simulink model "two_link_robot_dynamic_withoutg"  (R2020b)
settings: Solver=VariableStepAuto  StartTime=0.0  StopTime=10.0  RelTol=1e-3  EnableMultiTasking=on
undefined symbols (not defined in the file or in its folder): X, Y, Z
libraries: sm_lib x11, nesl_utility x11
settings Model: Creator=DELL  LastModifiedBy=Administrator
settings DataIOCC: LimitDataPoints=on  ReturnWorkspaceOutputs=off
settings OptimizationCC: LifeSpan=inf
settings DebuggingCC: AllowSymbolicDim=off  SFUnexpectedBacktrackingDiag=warning  SFNoUnconditionalDefaultTransitionDiag=warning  SFExecutionAtInitializationDiag=none  ArithmeticOperatorsInVariantConditions=warning
settings SFSimCC: SimUseLocalCustomCode=off  CustomCodeUndefinedFunction=UseInterfaceOnly
settings RTWCC: RTWUseLocalCustomCode=off
settings CodeAppCC: StateflowObjectComments=on
settings GRTTargetCC: TargetLangStandard=C89/C90 (ANSI)
settings ConfigComp: CovMetricSettings=dw  CovSaveCumulativeToWorkspaceVar=on  CovSaveSingleToWorkspaceVar=on  CovExternalEMLEnable=off  CovSFcnEnable=off
settings SimscapeCC: SimscapeNominalValues="[{\"value\":\"10\",\"unit\":\"V\"},{\"value\":\"1\",\"unit\":\"A\"},{\"value\":\"10\",\"unit\":\"N*m\"},{\"value\":\"10\",\"unit\":\"bar\"},{\"value\":\"100\",\"unit\":\"kJ/kg\"},{\"value\":\"1\",\"unit\":\"kW\"},{\"value\":\"300\",\"unit\":\"K\"},{\"value\":\"100\",\"unit\":\"cm^3/s\"},{\"value\":\"1\",\"unit\":\"kN\"},{\"value\":\"1\",\"unit\":\"g/cm^3\"},{\"value\":\"1\",\"unit\":\"l\"},{\"value\":\"1\",\"unit\":\"cm^2\"},{\"value\":\"60\",\"unit\":\"Hz\"}]"  SimscapeLogType=all  SimscapeLogDataHistory=10000
settings ConfigurationSet: Description=SimMechanics 2G

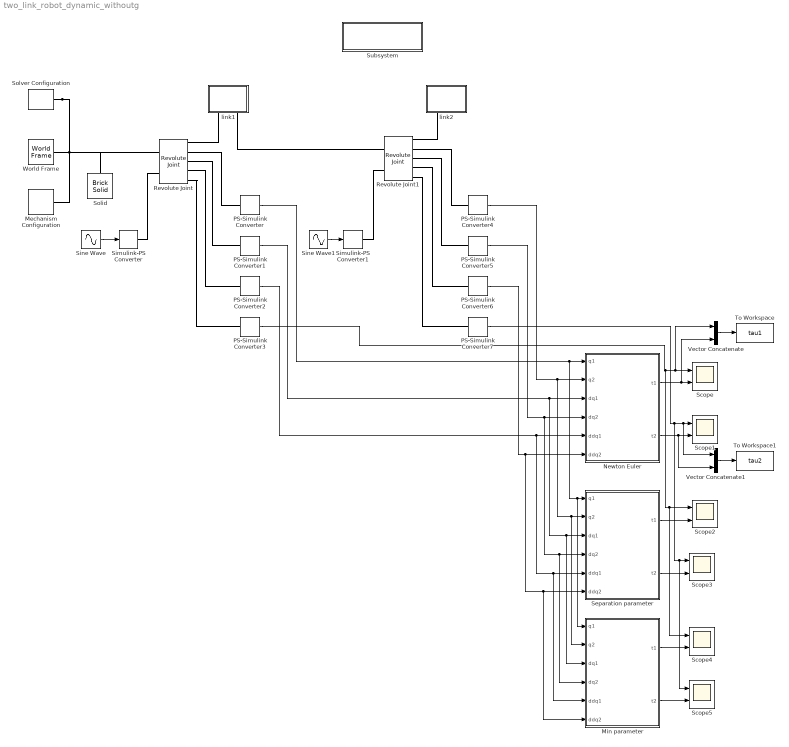
== system two_link_robot_dynamic_withoutg ==
  Mechanism Configuration : sm_lib/Utilities/Mechanism Configuration  UniformGravity=Constant  GravityVector=[0 0 0]  GravityVectorUnits=m/s^2  GravityUnits=m/s^2  LinearizationDelta=0.001  JointModeTransitionNonlinearIterations=2
  Min parameter : MATLAB Function  TreatAsAtomicUnit=on
  Newton Euler : MATLAB Function  TreatAsAtomicUnit=on
  PS-Simulink Converter{,1..7} (8 alike) : nesl_utility/PS-Simulink Converter  PhysicalDomain=network_engine_domain  SubClassName=ps_output  LeftPortType=input  RightPortType=output  PseudoPeriodic=off  Frequencies=[]  Unit=1  AffineConversion=off
  Revolute Joint : sm_lib/Joints/Revolute Joint  JointMode=Normal  SenseConstraintForce=off  SenseConstraintForceX=off  SenseConstraintForceY=off  SenseConstraintForceZ=off  SenseConstraintTorque=off  SenseConstraintTorqueX=off  SenseConstraintTorqueY=off  SenseConstraintTorqueZ=off  SenseTotalForce=off  SenseTotalForceX=off  SenseTotalForceY=off  SenseTotalForceZ=off  SenseTotalTorque=off  SenseTotalTorqueX=off  SenseTotalTorqueY=off  SenseTotalTorqueZ=off  CompositeWrenchDir=FollowerOnBase  CompositeWrenchFrame=BaseFrame  EquilibriumPosition=0  EquilibriumPositionUnits=deg  SpringStiffness=0  SpringStiffnessUnits=N*m/deg  DampingCoefficient=0  DampingCoefficientUnits=N*m/(deg/s)  TorqueActuationMode=ComputedTorque  MotionActuationMode=InputMotion  SensePosition=on  SenseVelocity=on  SenseAcceleration=on  SenseTorqueForce=on  SenseLowerLimitTorqueForce=off  SenseUpperLimitTorqueForce=off  LowerLimitSpecify=off  LowerLimitBound=-90  LowerLimitBoundUnits=deg  LowerLimitStiffness=1e4  LowerLimitStiffnessUnits=N*m/deg  LowerLimitDamping=10  LowerLimitDampingUnits=N*m/(deg/s)  LowerLimitTransitionRegionWidth=0.1  LowerLimitTransitionRegionWidthUnits=deg  UpperLimitSpecify=off  UpperLimitBound=90  UpperLimitBoundUnits=deg  UpperLimitStiffness=1e4  UpperLimitStiffnessUnits=N*m/deg  UpperLimitDamping=10  UpperLimitDampingUnits=N*m/(deg/s)  UpperLimitTransitionRegionWidth=0.1  UpperLimitTransitionRegionWidthUnits=deg  PositionTargetSpecify=off  PositionTargetPriority=High  PositionTargetValue=0  PositionTargetValueUnits=deg  VelocityTargetSpecify=off  VelocityTargetPriority=High  VelocityTargetValue=0  VelocityTargetValueUnits=deg/s
  Revolute Joint1 : sm_lib/Joints/Revolute Joint  JointMode=Normal  SenseConstraintForce=off  SenseConstraintForceX=off  SenseConstraintForceY=off  SenseConstraintForceZ=off  SenseConstraintTorque=off  SenseConstraintTorqueX=off  SenseConstraintTorqueY=off  SenseConstraintTorqueZ=off  SenseTotalForce=off  SenseTotalForceX=off  SenseTotalForceY=off  SenseTotalForceZ=off  SenseTotalTorque=off  SenseTotalTorqueX=off  SenseTotalTorqueY=off  SenseTotalTorqueZ=off  CompositeWrenchDir=FollowerOnBase  CompositeWrenchFrame=BaseFrame  EquilibriumPosition=0  EquilibriumPositionUnits=deg  SpringStiffness=0  SpringStiffnessUnits=N*m/deg  DampingCoefficient=0  DampingCoefficientUnits=N*m/(deg/s)  TorqueActuationMode=ComputedTorque  MotionActuationMode=InputMotion  SensePosition=on  SenseVelocity=on  SenseAcceleration=on  SenseTorqueForce=on  SenseLowerLimitTorqueForce=off  SenseUpperLimitTorqueForce=off  LowerLimitSpecify=off  LowerLimitBound=-90  LowerLimitBoundUnits=deg  LowerLimitStiffness=1e4  LowerLimitStiffnessUnits=N*m/deg  LowerLimitDamping=10  LowerLimitDampingUnits=N*m/(deg/s)  LowerLimitTransitionRegionWidth=0.1  LowerLimitTransitionRegionWidthUnits=deg  UpperLimitSpecify=off  UpperLimitBound=90  UpperLimitBoundUnits=deg  UpperLimitStiffness=1e4  UpperLimitStiffnessUnits=N*m/deg  UpperLimitDamping=10  UpperLimitDampingUnits=N*m/(deg/s)  UpperLimitTransitionRegionWidth=0.1  UpperLimitTransitionRegionWidthUnits=deg  PositionTargetSpecify=off  PositionTargetPriority=High  PositionTargetValue=0  PositionTargetValueUnits=deg  VelocityTargetSpecify=off  VelocityTargetPriority=High  VelocityTargetValue=0  VelocityTargetValueUnits=deg/s
  Scope{,1..5} (6 alike) : Scope  NumInputPorts=2
  Separation parameter : MATLAB Function  TreatAsAtomicUnit=on
  Simulink-PS Converter : nesl_utility/Simulink-PS Converter  PhysicalDomain=network_engine_domain  SubClassName=ps_input  LeftPortType=input  RightPortType=output  PseudoPeriodic=off  Frequencies=[]  NoiseDistribution=none  NoiseParameters=[]  Unit=1  AffineConversion=off  FilteringAndDerivatives=filter  SimscapeFilterOrder=2  InputFilterTimeConstant=0.001  UdotUserProvided=0
  Simulink-PS Converter1 : nesl_utility/Simulink-PS Converter  PhysicalDomain=network_engine_domain  SubClassName=ps_input  LeftPortType=input  RightPortType=output  PseudoPeriodic=off  Frequencies=[]  NoiseDistribution=none  NoiseParameters=[]  Unit=1  AffineConversion=off  FilteringAndDerivatives=filter  SimscapeFilterOrder=2  InputFilterTimeConstant=0.001  UdotUserProvided=0
  Sine Wave : Sin  Amplitude=2  Frequency=2  SampleTime=0
  Sine Wave1 : Sin  Frequency=3  SampleTime=0
  Solid : sm_lib/Body Elements/Brick Solid  GraphicAmbientColor=[0.15 0.15 0.15 1.0]  BasedOnType=Density  BrickDimensions=[0.04 0.04 0.04]  BrickDimensionUnits=m  CenterOfMass=[0 0 0]  CenterOfMassUnits=m  GraphicDiffuseColor=[0.85 0.45 0]  Density=1000  DensityUnits=kg/m^3  DoExposeReferenceFrame=on  GraphicEmissiveColor=[0.0 0.0 0.0 1.0]  ExportEntireGeometry=off  SerializedFrames=<Frames/>  MarkerShape=Sphere  MarkerSize=10  GraphicType=FromGeometry  InertiaType=CalculateFromGeometry  Mass=1  MassUnits=kg  MomentsOfInertia=[1 1 1]  MomentsOfInertiaUnits=kg*m^2  GraphicOpacity=1.0  ProductsOfInertia=[0 0 0]  ProductsOfInertiaUnits=kg*m^2  GraphicShininess=75  GraphicSpecularColor=[0.5 0.5 0.5 1.0]  GraphicVisPropType=SimpleVisualProperties
  Solver Configuration : nesl_utility/Solver Configuration  PhysicalDomain=network_engine_domain  SubClassName=solver  LeftPortType=input  RightPortType=generic  Tones=[]  Harmonics=[]  SimulateNoise=off  Profile=off  UseLocalSampling=off  EnableSwitchedLinearOptims=on  FrequencyDomain=off  UseCCode=off  RelTol=0.001  AbsTol=1e-06  MinStep=1e-09  ToWorkspace=off  RevertToSquareIcSolve=off  NumHomotopyIterations=100  PhasorMode=off  PhasorModeNumHarmonics=1  DoDC=off  ResidualTolerance=1e-09  UseLocalSolver=off  LocalSolverChoice=NE_BACKWARD_EULER_ADVANCER  LocalSolverSampleTime=0.001  DoFixedCost=off  MaxNonlinIter=3  MaxModeIter=2  ComputeImpulses=off  ImpulseIterations=2  LinearAlgebra=Sparse  EquationFormulation=NE_TIME_EF  DelaysMemoryBudget=1024  AutomaticFiltering=on  FilteringTimeConstant=0.001  PartitionStorageMethod=AS_NEEDED  PartitionMemoryBudget=1024  PartitionMethod=FAST
  Subsystem : Subsystem
      settings: OpenFcn=open_system('sm_lib')
      mask Display: disp(sprintf('Open Simscape Multibody\nLibrary'));
  To Workspace : ToWorkspace  VariableName=tau1  SaveFormat=Timeseries  SampleTime=-1
  To Workspace1 : ToWorkspace  VariableName=tau2  SaveFormat=Timeseries  SampleTime=-1
  Vector Concatenate : Concatenate
  Vector Concatenate1 : Concatenate
  World Frame : sm_lib/Frames and Transforms/World Frame
  link1 : Subsystem  mask{r=0.01, l=0.3, rho=100000000, rgb=[0.2, 0.2, 0.8]}
      mask prompts: r "radius(m)"; l "length(m)"; rho "density(kg/m^3)"; rgb "Color[R G B]"
  link2 : Subsystem  mask{r=0.01, l=0.2, rho=200000000, rgb=[0.2, 0.2, 0.8]}
      mask prompts: r "radius(m)"; l "length(m)"; rho "density(kg/m^3)"; rgb "Color[R G B]"
  wires:
  Sine Wave/1 -> Simulink-PS Converter/1
  Sine Wave1/1 -> Simulink-PS Converter1/1
  PS-Simulink Converter/1 -> Min parameter/1(q1), Separation parameter/1(q1), Newton Euler/1(q1)
  PS-Simulink Converter4/1 -> Min parameter/2(q2), Separation parameter/2(q2), Newton Euler/2(q2)
  PS-Simulink Converter1/1 -> Min parameter/3(dq1), Separation parameter/3(dq1), Newton Euler/3(dq1)
  PS-Simulink Converter5/1 -> Min parameter/4(dq2), Separation parameter/4(dq2), Newton Euler/4(dq2)
  PS-Simulink Converter2/1 -> Min parameter/5(ddq1), Separation parameter/5(ddq1), Newton Euler/5(ddq1)
  PS-Simulink Converter6/1 -> Min parameter/6(ddq2), Separation parameter/6(ddq2), Newton Euler/6(ddq2)
  Newton Euler/1(t1) -> Vector Concatenate/2, Scope/2
  PS-Simulink Converter3/1 -> Scope4/1, Scope2/1, Vector Concatenate/1, Scope/1
  Newton Euler/2(t2) -> Scope1/2, Vector Concatenate1/2
  PS-Simulink Converter7/1 -> Scope5/1, Scope3/1, Vector Concatenate1/1, Scope1/1
  Vector Concatenate/1 -> To Workspace/1
  Vector Concatenate1/1 -> To Workspace1/1
  Separation parameter/1(t1) -> Scope2/2
  Separation parameter/2(t2) -> Scope3/2
  Min parameter/1(t1) -> Scope4/2
  Min parameter/2(t2) -> Scope5/2
  connections:
  Solver Configuration/RConn1 -- Solid/RConn1 -- Revolute Joint/LConn1 -- Mechanism Configuration/RConn1 -- World Frame/RConn1
  link1/RConn1 -- Revolute Joint/RConn1
  link1/RConn2 -- Revolute Joint1/LConn1
  Revolute Joint1/RConn1 -- link2/RConn1
  Simulink-PS Converter/RConn1 -- Revolute Joint/LConn2
  Simulink-PS Converter1/RConn1 -- Revolute Joint1/LConn2
  Revolute Joint/RConn2 -- PS-Simulink Converter/LConn1
  Revolute Joint/RConn3 -- PS-Simulink Converter1/LConn1
  Revolute Joint/RConn4 -- PS-Simulink Converter2/LConn1
  Revolute Joint/RConn5 -- PS-Simulink Converter3/LConn1
  Revolute Joint1/RConn2 -- PS-Simulink Converter4/LConn1
  Revolute Joint1/RConn3 -- PS-Simulink Converter5/LConn1
  Revolute Joint1/RConn4 -- PS-Simulink Converter6/LConn1
  Revolute Joint1/RConn5 -- PS-Simulink Converter7/LConn1

== system two_link_robot_dynamic_withoutg/Subsystem ==

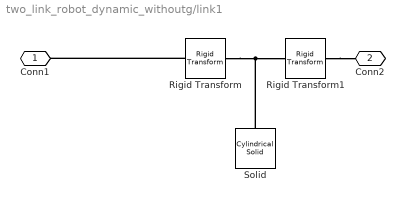
== system two_link_robot_dynamic_withoutg/link1 ==
  Rigid Transform : sm_lib/Frames and Transforms/Rigid Transform  TranslationMethod=StandardAxis  TranslationStandardOffset=l/2  TranslationLengthUnit=m  TranslationStandardAxis=-X  TranslationCartesianOffset=[0 0 0]  TranslationROffset=0  TranslationROffsetUnits=m  TranslationZOffset=0  TranslationZOffsetUnits=m  TranslationThetaOffset=0  TranslationThetaOffsetUnits=deg  RotationMethod=None  RotationAngleUnits=deg  RotationStandardAxis=-X  RotationAngle=0.0  RotationArbitraryAxis=[0 0 1]  FollAlignAxisA=+X  BaseAlignAxisA=+Y  FollAlignAxisB=+Y  BaseAlignAxisB=+Z  RotationSequenceAxes=FollowerAxes  RotationSequence=XYX  RotationSequenceAngles=[0 0 0]  RotationSequenceAnglesUnits=deg  RotationMatrix=[1 0 0; 0 1 0; 0 0 1]
  Rigid Transform1 : sm_lib/Frames and Transforms/Rigid Transform  TranslationMethod=StandardAxis  TranslationStandardOffset=l/2  TranslationLengthUnit=m  TranslationStandardAxis=+X  TranslationCartesianOffset=[0 0 0]  TranslationROffset=0  TranslationROffsetUnits=m  TranslationZOffset=0  TranslationZOffsetUnits=m  TranslationThetaOffset=0  TranslationThetaOffsetUnits=deg  RotationMethod=None  RotationAngleUnits=deg  RotationStandardAxis=+Z  RotationAngle=0.0  RotationArbitraryAxis=[0 0 1]  FollAlignAxisA=+X  BaseAlignAxisA=+Y  FollAlignAxisB=+Y  BaseAlignAxisB=+Z  RotationSequenceAxes=FollowerAxes  RotationSequence=XYX  RotationSequenceAngles=[0 0 0]  RotationSequenceAnglesUnits=deg  RotationMatrix=[1 0 0; 0 1 0; 0 0 1]
  Solid : sm_lib/Body Elements/Cylindrical Solid  GraphicAmbientColor=[0.15 0.15 0.15 1.0]  BasedOnType=Density  CenterOfMass=[0 0 0]  CenterOfMassUnits=m  GraphicDiffuseColor=rgb  CylinderLength=l  CylinderLengthUnits=m  CylinderRadius=r  CylinderRadiusUnits=m  Density=rho  DensityUnits=kg/m^3  DoExposeReferenceFrame=off  GraphicEmissiveColor=[0.0 0.0 0.0 1.0]  ExportEntireGeometry=off  SerializedFrames=<Frames><Frame><Id>Frame1</Id><Value><Name>F1</Name><Origin><Source>ReferenceFrame</Source><FeatureName></FeatureName></Origin><PrimaryAxis><DefinedDirection>+X</DefinedDirection><Source>ReferenceFrame</Source><SourceDirection>+Z</SourceDirection><FeatureName></FeatureName></PrimaryAxis><SecondaryAxis><DefinedDirection>+Y</DefinedDirection><Source>ReferenceFrame</Source><SourceDirection>+X</SourceDirection><FeatureName></FeatureName></SecondaryAxis></Value></Frame></Frames>  MarkerShape=Sphere  MarkerSize=10  GraphicType=FromGeometry  InertiaType=CalculateFromGeometry  Mass=1  MassUnits=kg  MomentsOfInertia=[1 1 1]  MomentsOfInertiaUnits=kg*m^2  GraphicOpacity=1.0  ProductsOfInertia=[0 0 0]  ProductsOfInertiaUnits=kg*m^2  GraphicShininess=75  GraphicSpecularColor=[0.5 0.5 0.5 1.0]  GraphicVisPropType=SimpleVisualProperties
  Conn1 : PMIOPort  Side=Right
  Conn2 : PMIOPort  Port=2  Side=Right
  connections:
  Rigid Transform/LConn1 -- Rigid Transform1/LConn1 -- Solid/LConn1
  Rigid Transform1/RConn1 -- Conn2/RConn1
  Rigid Transform/RConn1 -- Conn1/RConn1

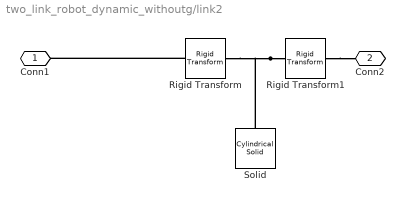
== system two_link_robot_dynamic_withoutg/link2 ==
  Rigid Transform : sm_lib/Frames and Transforms/Rigid Transform  TranslationMethod=StandardAxis  TranslationStandardOffset=l/2  TranslationLengthUnit=m  TranslationStandardAxis=-X  TranslationCartesianOffset=[0 0 0]  TranslationROffset=0  TranslationROffsetUnits=m  TranslationZOffset=0  TranslationZOffsetUnits=m  TranslationThetaOffset=0  TranslationThetaOffsetUnits=deg  RotationMethod=None  RotationAngleUnits=deg  RotationStandardAxis=-X  RotationAngle=0.0  RotationArbitraryAxis=[0 0 1]  FollAlignAxisA=+X  BaseAlignAxisA=+Y  FollAlignAxisB=+Y  BaseAlignAxisB=+Z  RotationSequenceAxes=FollowerAxes  RotationSequence=XYX  RotationSequenceAngles=[0 0 0]  RotationSequenceAnglesUnits=deg  RotationMatrix=[1 0 0; 0 1 0; 0 0 1]
  Rigid Transform1 : sm_lib/Frames and Transforms/Rigid Transform  TranslationMethod=StandardAxis  TranslationStandardOffset=l/2  TranslationLengthUnit=m  TranslationStandardAxis=+X  TranslationCartesianOffset=[0 0 0]  TranslationROffset=0  TranslationROffsetUnits=m  TranslationZOffset=0  TranslationZOffsetUnits=m  TranslationThetaOffset=0  TranslationThetaOffsetUnits=deg  RotationMethod=None  RotationAngleUnits=deg  RotationStandardAxis=+Z  RotationAngle=0.0  RotationArbitraryAxis=[0 0 1]  FollAlignAxisA=+X  BaseAlignAxisA=+Y  FollAlignAxisB=+Y  BaseAlignAxisB=+Z  RotationSequenceAxes=FollowerAxes  RotationSequence=XYX  RotationSequenceAngles=[0 0 0]  RotationSequenceAnglesUnits=deg  RotationMatrix=[1 0 0; 0 1 0; 0 0 1]
  Solid : sm_lib/Body Elements/Cylindrical Solid  GraphicAmbientColor=[0.15 0.15 0.15 1.0]  BasedOnType=Density  CenterOfMass=[0 0 0]  CenterOfMassUnits=m  GraphicDiffuseColor=rgb  CylinderLength=l  CylinderLengthUnits=m  CylinderRadius=r  CylinderRadiusUnits=m  Density=rho  DensityUnits=kg/m^3  DoExposeReferenceFrame=off  GraphicEmissiveColor=[0.0 0.0 0.0 1.0]  ExportEntireGeometry=off  SerializedFrames=<Frames><Frame><Id>Frame1</Id><Value><Name>F1</Name><Origin><Source>ReferenceFrame</Source><FeatureName></FeatureName></Origin><PrimaryAxis><DefinedDirection>+X</DefinedDirection><Source>ReferenceFrame</Source><SourceDirection>+Z</SourceDirection><FeatureName></FeatureName></PrimaryAxis><SecondaryAxis><DefinedDirection>+Y</DefinedDirection><Source>ReferenceFrame</Source><SourceDirection>+X</SourceDirection><FeatureName></FeatureName></SecondaryAxis></Value></Frame></Frames>  MarkerShape=Sphere  MarkerSize=10  GraphicType=FromGeometry  InertiaType=CalculateFromGeometry  Mass=1  MassUnits=kg  MomentsOfInertia=[1 1 1]  MomentsOfInertiaUnits=kg*m^2  GraphicOpacity=1.0  ProductsOfInertia=[0 0 0]  ProductsOfInertiaUnits=kg*m^2  GraphicShininess=75  GraphicSpecularColor=[0.5 0.5 0.5 1.0]  GraphicVisPropType=SimpleVisualProperties
  Conn1 : PMIOPort  Side=Right
  Conn2 : PMIOPort  Port=2  Side=Right
  connections:
  Rigid Transform/RConn1 -- Conn1/RConn1
  Rigid Transform1/RConn1 -- Conn2/RConn1
  Rigid Transform1/LConn1 -- Rigid Transform/LConn1 -- Solid/LConn1

== matlab function two_link_robot_dynamic_withoutg/Separation parameter ==
  data: q1 input; t1 output; q2 input; dq1 input; dq2 input; ddq1 input; ddq2 input; t2 output
function [t1,t2] = fcn(q1,q2,dq1,dq2,ddq1,ddq2)
%连杆1质心惯性张量
L_1xx = 0.471239;
L_1xy = 0;
L_1xz = 0;
L_1yy = 70.9215;
L_1yz = 0;
L_1zz = 70.9215;
m_1 = 9424.78;
L_1c = [L_1xx 0 0;0 L_1yy 0;0 0 L_1zz];
%连杆2质心惯性张量
L_2xx = 0.628319;
L_2xy = 0;
L_2xz = 0;
L_2yy = 42.2021;
L_2yz = 0;
L_2zz = 42.2021;
m_2 = 12566.4;
L_2c = [L_2xx 0 0;0 L_2yy 0;0 0 L_2zz];
%连杆长度
l1 = 0.3;
l2 = 0.2;
%质心坐标
l_1x = l1 / 2;
l_1y = 0;
l_1z = 0;
pc1 = [l_1x l_1y l_1z]';
l_2x = l2 / 2;
l_2y = 0;
l_2z = 0;
pc2 = [l_2x l_2y l_2z]';
%平行轴定理，旋转轴处的惯性张量
I3 = eye(3);
L_1 = L_1c + m_1*(pc1'*pc1*I3 - pc1*pc1');
L_2 = L_2c + m_2*(pc2'*pc2*I3 - pc2*pc2');

% 地杆角速度
w_0_0 = [0;0;0];
% 地杆线速度速度
v_0_0 = [0;0;0];
% angular acceleration of base link
alpha_0_0 = [0; 0; 0];
% 考虑重力，初始加速度y0方向
% a_0_0 = [0; 9.81; 0];
a_0_0 = [0; 0; 0];

dh = [0, 0, 0, q1;
      0, l1, 0, q2];

w = cell(1, size(dh, 1));
v = cell(1, size(dh, 1));
alpha = cell(1, size(dh, 1));
a = cell(1, size(dh, 1));
ac = cell(1, size(dh, 1));
l = cell(1, size(dh, 1));
T = cell(1, size(dh, 1) + 1);
R = cell(1, size(dh, 1) + 1);
r = cell(1, size(dh, 1) + 1);
I = cell(1, size(dh, 1));
T_e = cell(1, size(dh, 1) + 1);
t_e_pre = eye(4);
for i = 1:size(dh, 1)
    trx = [1 0 0 0; 
           0 cos(dh(i, 1)) -sin(dh(i, 1)) 0;
           0 sin(dh(i, 1)) cos(dh(i, 1))  0;
           0 0 0 1];
    tl = [1 0 0 dh(i, 2);
          0 1 0 0;
          0 0 1 dh(i, 3);
          0 0 0 1];
    trz = [cos(dh(i, 4)) -sin(dh(i, 4)) 0 0;
           sin(dh(i, 4)) cos(dh(i, 4))  0 0;
           0 0 1 0;
           0 0 0 1];
    T{i} = trx * tl * trz;%trotx(dh(i, 1))*transl([dh(i, 2), 0, dh(i, 3)])*trotz(dh(i, 4));
    R{i} = T{i}(1:3, 1:3);
    r{i} = T{i}(1:3, 4);
    T_e{i} = t_e_pre * T{i};
    t_e_pre = T_e{i};
end
T{i+1} = eye(3);
R{i+1} = eye(3);
r{i+1} = [l2, 0, 0];
T_e{i+1} = T_e{i} * [1 0 0 l2; 0 1 0 0; 0 0 1 0; 0 0 0 1];%T_e{i} * transl([l2, 0, 0]);
q = [q1 q2];
dq = [dq1 dq2];
ddq = [ddq1 ddq2];
l{1} = [l_1x; l_1y; l_1z];
l{2} = [l_2x; l_2y; l_2z];

pre_w = w_0_0;
pre_v = v_0_0;
pre_alpha = alpha_0_0;
pre_a = a_0_0;
% 外推
for i = 1:2
    t = R{i}';
    w_i_i = t * pre_w + dq(i) * [0;0;1];
    v_i_i = t * (pre_v + cross(pre_w, r{i}));
    alpha_i_i = t * pre_alpha + cross((t * pre_w), dq(i) * [0;0;1]) + ddq(i) * [0;0;1];
    a_i_i = t * (pre_a + cross(pre_alpha, r{i}) + cross(pre_w, cross(pre_w, r{i})));
    ac_i_i = a_i_i + cross(alpha_i_i, l{i}) + cross(w_i_i, cross(w_i_i, l{i}));
    w{i} = w_i_i;
    v{i} = v_i_i;
    alpha{i} = alpha_i_i;
    a{i} = a_i_i;
    ac{i} = ac_i_i;
    
    pre_w = w_i_i;
    pre_v = v_i_i;
    pre_alpha = alpha_i_i;
    pre_a = a_i_i;
end

%参数分离参数
A1 = zeros(6,10);
A2 = zeros(6,10);
A1(1:3,1) = a{1};
A1(1:3,2:4) = S_alg(alpha{1})+S_alg(w{1})*S_alg(w{1});
A1(4:6,2:4) = -S_alg(a{1});
A1(4:6,5:10) = K_alg(alpha{1})+S_alg(w{1})*K_alg(w{1});
A2(1:3,1) = a{2};
A2(1:3,2:4) = S_alg(alpha{2})+S_alg(w{2})*S_alg(w{2});
A2(4:6,2:4) = -S_alg(a{2});
A2(4:6,5:10) = K_alg(alpha{2})+S_alg(w{2})*K_alg(w{2});

R21 = R{2};
P21 = r{2};
Q12 = [R21 zeros(3,3);S_alg(P21)*R21 R21];
U11 = A1;
U12 = Q12*A2;
U22 = A2; 
U1 = [U11 U12;
zeros(6,10) U22]; 
U = [U1(6,:);
 U1(12,:);]; 
%     
fi1 = [m_1 m_1*l_1x m_1*l_1y m_1*l_1z L_1(1,1) -L_1(1,2) -L_1(1,3) L_1(2,2) -L_1(2,3) L_1(3,3)]';
fi2  = [m_2 m_2*l_2x m_2*l_2y m_2*l_2z L_2(1,1) -L_2(1,2) -L_2(1,3) L_2(2,2) -L_2(2,3) L_2(3,3)]';
fi = [fi1;fi2]; %线性分离的  
f = U1*fi;
t1 = f(6);
t2 = f(12);
end

function T = K_alg(w)
 wx = w(1);wy = w(2);wz = w(3);
 T = zeros(3,6);
 T(1,1) = wx;T(1,2) = wy;T(1,3) = wz;
 T(2,2) = wx;T(2,4) = wy;T(2,5) = wz;
 T(3,3) = wx;T(3,5) = wy;T(3,6) = wz;
end

function T = S_alg(w)
 w_r = eye(3);
 A1 = w(1);A2 = w(2);A3 = w(3);
 w_r(1,1) = 0;w_r(1,2) = -A3;w_r(1,3) = A2;
 w_r(2,1) = A3;w_r(2,2) = 0;w_r(2,3) = -A1;
 w_r(3,1) = -A2;w_r(3,2) = A1;w_r(3,3) = 0;
 T = w_r;
end

== matlab function two_link_robot_dynamic_withoutg/Newton Euler ==
  data: q1 input; t1 output; q2 input; dq1 input; dq2 input; ddq1 input; ddq2 input; t2 output
function [t1,t2] = fcn(q1,q2,dq1,dq2,ddq1,ddq2)
%连杆1质心惯性张量
L_1xx = 0.471239;
L_1xy = 0;
L_1xz = 0;
L_1yy = 70.9215;
L_1yz = 0;
L_1zz = 70.9215;
m_1 = 9424.78;
L_1c = [L_1xx 0 0;0 L_1yy 0;0 0 L_1zz];
%连杆2质心惯性张量
L_2xx = 0.628319;
L_2xy = 0;
L_2xz = 0;
L_2yy = 42.2021;
L_2yz = 0;
L_2zz = 42.2021;
m_2 = 12566.4;
L_2c = [L_2xx 0 0;0 L_2yy 0;0 0 L_2zz];
%连杆长度
l1 = 0.3;
l2 = 0.2;
%质心坐标
l_1x = l1 / 2;
l_1y = 0;
l_1z = 0;
pc1 = [l_1x l_1y l_1z]';
l_2x = l2 / 2;
l_2y = 0;
l_2z = 0;
pc2 = [l_2x l_2y l_2z]';
%平行轴定理，旋转轴处的惯性张量
I3 = eye(3);
L_1 = L_1c + m_1*(pc1'*pc1*I3 - pc1*pc1');
L_2 = L_2c + m_2*(pc2'*pc2*I3 - pc2*pc2');

% 地杆角速度
w_0_0 = [0;0;0];
% 地杆线速度速度
v_0_0 = [0;0;0];
% angular acceleration of base link
alpha_0_0 = [0; 0; 0];
% 不考虑重力
% a_0_0 = [0; 9.81; 0];
a_0_0 = [0; 0; 0];

dh = [0, 0, 0, q1;
      0, l1, 0, q2];

w = cell(1, size(dh, 1));
v = cell(1, size(dh, 1));
alpha = cell(1, size(dh, 1));
a = cell(1, size(dh, 1));
ac = cell(1, size(dh, 1));
l = cell(1, size(dh, 1));
T = cell(1, size(dh, 1) + 1);
R = cell(1, size(dh, 1) + 1);
r = cell(1, size(dh, 1) + 1);
I = cell(1, size(dh, 1));
T_e = cell(1, size(dh, 1) + 1);
t_e_pre = eye(4);
for i = 1:size(dh, 1)
    trx = [1 0 0 0; 
           0 cos(dh(i, 1)) -sin(dh(i, 1)) 0;
           0 sin(dh(i, 1)) cos(dh(i, 1))  0;
           0 0 0 1];
    tl = [1 0 0 dh(i, 2);
          0 1 0 0;
          0 0 1 dh(i, 3);
          0 0 0 1];
    trz = [cos(dh(i, 4)) -sin(dh(i, 4)) 0 0;
           sin(dh(i, 4)) cos(dh(i, 4))  0 0;
           0 0 1 0;
           0 0 0 1];
    T{i} = trx * tl * trz;%trotx(dh(i, 1))*transl([dh(i, 2), 0, dh(i, 3)])*trotz(dh(i, 4));其次变换矩阵
    R{i} = T{i}(1:3, 1:3);
    r{i} = T{i}(1:3, 4);
    T_e{i} = t_e_pre * T{i};
    t_e_pre = T_e{i};
end
T{i+1} = eye(3);
R{i+1} = eye(3);
r{i+1} = [l2, 0, 0];
T_e{i+1} = T_e{i} * [1 0 0 l2; 0 1 0 0; 0 0 1 0; 0 0 0 1];%T_e{i} * transl([l2, 0, 0]);
q = [q1 q2];
dq = [dq1 dq2];
ddq = [ddq1 ddq2];
l{1} = [l_1x; l_1y; l_1z];
l{2} = [l_2x; l_2y; l_2z];

pre_w = w_0_0;
pre_v = v_0_0;
pre_alpha = alpha_0_0;
pre_a = a_0_0;
% 外推
for i = 1:2
    t = R{i}';
    w_i_i = t * pre_w + dq(i) * [0;0;1];
    v_i_i = t * (pre_v + cross(pre_w, r{i}));
    alpha_i_i = t * pre_alpha + cross((t * pre_w), dq(i) * [0;0;1]) + ddq(i) * [0;0;1];
    a_i_i = t * (pre_a + cross(pre_alpha, r{i}) + cross(pre_w, cross(pre_w, r{i})));
    ac_i_i = a_i_i + cross(alpha_i_i, l{i}) + cross(w_i_i, cross(w_i_i, l{i}));
    w{i} = w_i_i;
    v{i} = v_i_i;
    alpha{i} = alpha_i_i;
    a{i} = a_i_i;
    ac{i} = ac_i_i;
    
    pre_w = w_i_i;
    pre_v = v_i_i;
    pre_alpha = alpha_i_i;
    pre_a = a_i_i;
end
m = [m_1; m_2];
% 内推
f_3_3 = [0;0;0];
n_3_3 = [0;0;0];
next_f_i_i = f_3_3;
next_n_i_i = n_3_3;

I{1} = [L_1xx L_1xy L_1xz; L_1xy L_1yy L_1yz; L_1xz L_1yz L_1zz];
I{2} = [L_2xx L_2xy L_2xz; L_2xy L_2yy L_2yz; L_2xz L_2yz L_2zz];
tau = cell(1, size(dh, 1));

for i = 2:-1:1
    rr = R{i+1};
    f_i_i = m(i)*ac{i} + rr * next_f_i_i;
    
    TT = T_e{i};
    TT(1:3,1:3) = (T_e{i}(1:3,1:3))';
    TT(1:3, 4) = -(T_e{i}(1:3,1:3))' * T_e{i}(1:3,4);
    xx = TT * T_e{i+1}(1:4, 4);
    r_ip1_ci = l{i} - xx(1:3);
    torque_i = I{i}*alpha{i} + cross(w{i}, I{i}*w{i}) + rr * next_n_i_i + cross(l{i}, f_i_i) - cross(r_ip1_ci, rr * next_f_i_i);
    tau{i} = torque_i(3);
    next_f_i_i = f_i_i;
    next_n_i_i = torque_i;
end
t1 = tau{1};
t2 = tau{2};


end

== matlab function two_link_robot_dynamic_withoutg/Min parameter ==
  data: q1 input; t1 output; q2 input; dq1 input; dq2 input; ddq1 input; ddq2 input; t2 output
function [t1,t2] = fcn(q1,q2,dq1,dq2,ddq1,ddq2)
%连杆1质心惯性张量
L_1xx = 0.471239;
L_1xy = 0;
L_1xz = 0;
L_1yy = 70.9215;
L_1yz = 0;
L_1zz = 70.9215;
m_1 = 9424.78;
L_1c = [L_1xx 0 0;0 L_1yy 0;0 0 L_1zz];
%连杆2质心惯性张量
L_2xx = 0.628319;
L_2xy = 0;
L_2xz = 0;
L_2yy = 42.2021;
L_2yz = 0;
L_2zz = 42.2021;
m_2 = 12566.4;
L_2c = [L_2xx 0 0;0 L_2yy 0;0 0 L_2zz];
%连杆长度
l1 = 0.3;
l2 = 0.2;
%质心坐标
l_1x = l1 / 2;
l_1y = 0;
l_1z = 0;
pc1 = [l_1x l_1y l_1z]';
l_2x = l2 / 2;
l_2y = 0;
l_2z = 0;
pc2 = [l_2x l_2y l_2z]';
%平行轴定理，旋转轴处的惯性张量
I3 = eye(3);
L_1 = L_1c + m_1*(pc1'*pc1*I3 - pc1*pc1');
L_2 = L_2c + m_2*(pc2'*pc2*I3 - pc2*pc2');

% 地杆角速度
w_0_0 = [0;0;0];
% 地杆线速度速度
v_0_0 = [0;0;0];
% angular acceleration of base link
alpha_0_0 = [0; 0; 0];
% 不考虑重力
% a_0_0 = [0; 9.81; 0];
a_0_0 = [0; 0; 0];

dh = [0, 0, 0, q1;
      0, l1, 0, q2];

w = cell(1, size(dh, 1));
v = cell(1, size(dh, 1));
alpha = cell(1, size(dh, 1));
a = cell(1, size(dh, 1));
ac = cell(1, size(dh, 1));
l = cell(1, size(dh, 1));
T = cell(1, size(dh, 1) + 1);
R = cell(1, size(dh, 1) + 1);
r = cell(1, size(dh, 1) + 1);
I = cell(1, size(dh, 1));
T_e = cell(1, size(dh, 1) + 1);
t_e_pre = eye(4);
for i = 1:size(dh, 1)
    trx = [1 0 0 0; 
           0 cos(dh(i, 1)) -sin(dh(i, 1)) 0;
           0 sin(dh(i, 1)) cos(dh(i, 1))  0;
           0 0 0 1];
    tl = [1 0 0 dh(i, 2);
          0 1 0 0;
          0 0 1 dh(i, 3);
          0 0 0 1];
    trz = [cos(dh(i, 4)) -sin(dh(i, 4)) 0 0;
           sin(dh(i, 4)) cos(dh(i, 4))  0 0;
           0 0 1 0;
           0 0 0 1];
    T{i} = trx * tl * trz;%trotx(dh(i, 1))*transl([dh(i, 2), 0, dh(i, 3)])*trotz(dh(i, 4));其次变换矩阵
    R{i} = T{i}(1:3, 1:3);
    r{i} = T{i}(1:3, 4);
    T_e{i} = t_e_pre * T{i};
    t_e_pre = T_e{i};
end
T{i+1} = eye(3);
R{i+1} = eye(3);
r{i+1} = [l2, 0, 0];
T_e{i+1} = T_e{i} * [1 0 0 l2; 0 1 0 0; 0 0 1 0; 0 0 0 1];%T_e{i} * transl([l2, 0, 0]);
q = [q1 q2];
dq = [dq1 dq2];
ddq = [ddq1 ddq2];
l{1} = [l_1x; l_1y; l_1z];
l{2} = [l_2x; l_2y; l_2z];

pre_w = w_0_0;
pre_v = v_0_0;
pre_alpha = alpha_0_0;
pre_a = a_0_0;
% 外推
for i = 1:2
    t = R{i}';
    w_i_i = t * pre_w + dq(i) * [0;0;1];
    v_i_i = t * (pre_v + cross(pre_w, r{i}));
    alpha_i_i = t * pre_alpha + cross((t * pre_w), dq(i) * [0;0;1]) + ddq(i) * [0;0;1];
    a_i_i = t * (pre_a + cross(pre_alpha, r{i}) + cross(pre_w, cross(pre_w, r{i})));
    ac_i_i = a_i_i + cross(alpha_i_i, l{i}) + cross(w_i_i, cross(w_i_i, l{i}));
    w{i} = w_i_i;
    v{i} = v_i_i;
    alpha{i} = alpha_i_i;
    a{i} = a_i_i;
    ac{i} = ac_i_i;
    
    pre_w = w_i_i;
    pre_v = v_i_i;
    pre_alpha = alpha_i_i;
    pre_a = a_i_i;
end

%参数分离参数
A1 = zeros(6,10);
A2 = zeros(6,10);
A1(1:3,1) = a{1};
A1(1:3,2:4) = S_alg(alpha{1})+S_alg(w{1})*S_alg(w{1});
A1(4:6,2:4) = -S_alg(a{1});
A1(4:6,5:10) = K_alg(alpha{1})+S_alg(w{1})*K_alg(w{1});
A2(1:3,1) = a{2};
A2(1:3,2:4) = S_alg(alpha{2})+S_alg(w{2})*S_alg(w{2});
A2(4:6,2:4) = -S_alg(a{2});
A2(4:6,5:10) = K_alg(alpha{2})+S_alg(w{2})*K_alg(w{2});

R21 = R{2};
P21 = r{2};
Q12 = [R21 zeros(3,3);S_alg(P21)*R21 R21];
U11 = A1;
U12 = Q12*A2;
U22 = A2; 
U1 = [U11 U12;
zeros(6,10) U22]; 
U = [U1(6,:);
 U1(12,:);]; 
    
fi1 = [m_1 m_1*l_1x m_1*l_1y m_1*l_1z L_1(1,1) -L_1(1,2) -L_1(1,3) L_1(2,2) -L_1(2,3) L_1(3,3)]';
fi2  = [m_2 m_2*l_2x m_2*l_2y m_2*l_2z L_2(1,1) -L_2(1,2) -L_2(1,3) L_2(2,2) -L_2(2,3) L_2(3,3)]';
%init
M2 = fi2(1,1);
MX2 = fi2(2,1);
MY2 = fi2(3,1);
MZ2 = fi2(4,1);
XX2 = fi2(5,1);
XY2 = fi2(6,1);
XZ2 = fi2(7,1);
YY2 = fi2(8,1);
YZ2 = fi2(9,1);
ZZ2 = fi2(10,1);
%r2
fi2_min_param = [MX2 MY2 ZZ2]';

d2 = 0;
a2 = l1;
alpha2 = 0;
cs2 = cos(alpha2)*sin(alpha2);
s2 = sin(alpha2);
c2 = cos(alpha2);

XX1 = fi1(5,1) + d2^2*M2;
XY1 = fi1(6,1) + a2*d2*s2*M2;
XZ1 = fi1(7,1) - a2*d2*c2*M2;
YY1 = fi1(8,1) + (a2^2 + d2^2*c2^2)*M2;
YZ1 = fi1(9,1) + d2^2*cs2*M2; 
ZZ1 = fi1(10,1) + (a2^2 + d2^2*s2^2)*M2;
MX1 = fi1(2,1) + a2*M2;
MY1 = fi1(3,1) - d2*s2*M2;
MZ1 = fi1(4,1) + d2*c2*M2;
M1 = fi1(1,1) + M2;

%r3
%不考虑重力
% fi1_min_param = [MX1 ZZ1]';
fi1_min_param =  ZZ1;
fi_min_param = [fi1_min_param;fi2_min_param];  
% U_min_param = zeros(2,5);
% U_min_param(:,1) = U(:,2);
% U_min_param(:,2) = U(:,10);
% U_min_param(:,3) = U(:,12);
% U_min_param(:,4) = U(:,13);
% U_min_param(:,5) = U(:,20);
U_min_param = zeros(2,4);
U_min_param(:,1) = U(:,10);
U_min_param(:,2) = U(:,12);
U_min_param(:,3) = U(:,13);
U_min_param(:,4) = U(:,20);
tao = U_min_param*fi_min_param;

t1 = tao(1);
t2 = tao(2); 
end

function T = K_alg(w)
 wx = w(1);wy = w(2);wz = w(3);
 T = zeros(3,6);
 T(1,1) = wx;T(1,2) = wy;T(1,3) = wz;
 T(2,2) = wx;T(2,4) = wy;T(2,5) = wz;
 T(3,3) = wx;T(3,5) = wy;T(3,6) = wz;
end

function T = S_alg(w)
 w_r = eye(3);
 A1 = w(1);A2 = w(2);A3 = w(3);
 w_r(1,1) = 0;w_r(1,2) = -A3;w_r(1,3) = A2;
 w_r(2,1) = A3;w_r(2,2) = 0;w_r(2,3) = -A1;
 w_r(3,1) = -A2;w_r(3,2) = A1;w_r(3,3) = 0;
 T = w_r;
end
